simulink model "Sliding_Mode2"  (R2020b)
settings: Solver=VariableStepAuto  StartTime=0.0  StopTime=15  RelTol=1e-3
settings Model: Creator=zhiyao  LastModifiedBy=zhiyao

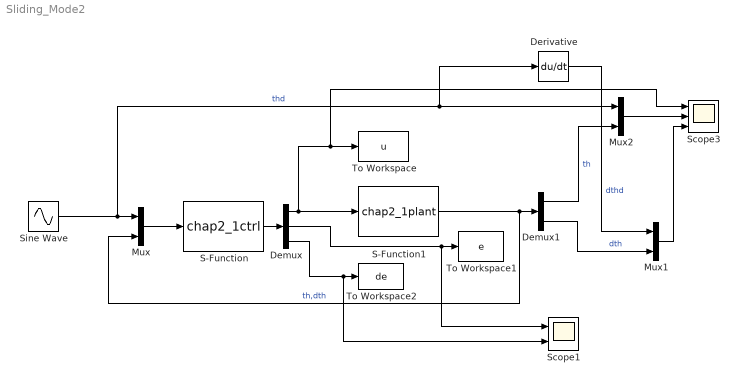
== system Sliding_Mode2 ==
  Demux : Demux  Outputs=3
  Demux1 : Demux  Outputs=2
  Derivative : Derivative
  Mux : Mux  Inputs=2
  Mux1 : Mux  Inputs=2
  Mux2 : Mux  Inputs=2
  S-Function : S-Function  FunctionName=chap2_1ctrl  SFunctionDeploymentMode=off  EnableBusSupport=off
  S-Function1 : S-Function  FunctionName=chap2_1plant  SFunctionDeploymentMode=off  EnableBusSupport=off
  Scope1 : Scope  NumInputPorts=2
  Scope3 : Scope  NumInputPorts=3
  Sine Wave : Sin  SampleTime=0
  To Workspace : ToWorkspace  VariableName=u  SaveFormat=Timeseries  SampleTime=-1
  To Workspace1 : ToWorkspace  VariableName=e  SaveFormat=Timeseries  SampleTime=-1
  To Workspace2 : ToWorkspace  VariableName=de  SaveFormat=Timeseries  SampleTime=-1
  wires:
  Mux/1 -> S-Function/1
  Sine Wave/1 -> Derivative/1, Mux2/1, Mux/1  "thd"
  S-Function/1 -> Demux/1
  Demux/1 -> S-Function1/1, Scope3/1, To Workspace/1
  Demux/2 -> Scope1/1, To Workspace1/1
  Demux/3 -> Scope1/2, To Workspace2/1
  S-Function1/1 -> Demux1/1, Mux/2  "th,dth"
  Mux2/1 -> Scope3/2
  Demux1/1 -> Mux2/2  "th"
  Mux1/1 -> Scope3/3
  Demux1/2 -> Mux1/2  "dth"
  Derivative/1 -> Mux1/1  "dthd"
